simulink model "EmbeddedClosedLoop_Ard"  (Simulink 10.0)
settings: Solver=ode3  StartTime=0.0  StopTime=10.0  RelTol=1e-3
libraries: arduinolib x5, simulink x3
settings Model: Creator=deastman  LastModifiedBy=bhisma  ExtModeTrigDuration=2
settings DataIOCC: LimitDataPoints=on  SignalLoggingSaveFormat=ModelDataLogs
settings OptimizationCC: ExpressionDepthLimit=2147483647  LifeSpan=1  EfficientTunableParamExpr=on
settings DebuggingCC: FcnCallInpInsideContextMsg=warning  StateNameClashWarn=warning
settings HardwareCC: ProdBitPerInt=16  ProdBitPerPointer=16  ProdBitPerSizeT=16  ProdBitPerPtrDiffT=16  ProdIntDivRoundTo=Zero  ProdEndianess=LittleEndian  ProdWordSize=8  ProdHWDeviceType=Atmel->AVR
settings SFSimCC: MATLABDynamicMemAlloc=off
settings RTWCC: Description=Real-Time Toolbox  SystemTargetFile=realtime.tlc  GenerateMakefile=off  TemplateMakefile=realtime.tmf  RTWVerbose=off
settings CodeAppCC: CustomSymbolStrType=$N$R$M  InternalIdentifier=Classic
settings STFCustomTargetCC: TargetLibSuffix=.a  GenerateSampleERTMain=on  ERTCustomFileBanners=on  SupportNonInlinedSFcns=off  RemoveResetFunc=on  SupportVariableSizeSignals=on  MATLABClassNameForMDSCustomization=Simulink.SoftwareTarget.ERTCustomization  GRTInterface=off  SystemTargetFile=realtime.tlc
settings ERTTargetCC: MultiwordLength=2048  GenerateSampleERTMain=on  ParMdlRefBuildCompliant=off  CompOptLevelCompliant=off  ConcurrentExecutionCompliant=off  CombineOutputUpdateFcns=off  SupportContinuousTime=on  SupportVariableSizeSignals=on  ModelStepFunctionPrototypeControlCompliant=off  CPPClassGenCompliant=off  UseToolchainInfoCompliant=off  ERTSrcFileBannerTemplate=realtime_code_template.cgt  ERTHdrFileBannerTemplate=realtime_code_template.cgt  ERTDataSrcFileTemplate=realtime_code_template.cgt  ERTDataHdrFileTemplate=realtime_code_template.cgt  ERTCustomFileTemplate=realtime_file_process.tlc  ConvertIfToSwitch=off  SuppressUnreachableDefaultCases=off
settings ConfigComp: CovExternalEMLEnable=off
settings SimscapeCC: SimscapeNormalizeSystem=off
settings ConfigurationSet: Description=SimMechanics 2G
settings SettingsController: Description=Run on Hardware Dialog  TargetExtensionPlatform=Arduino Uno
settings MATStruct: Set_host_COM_port=[0.0]  COM_port_number=1  COM_port_baud_rate=115200  Enable_overrun_detection=[0.0]  Digital_output_to_set_on_overrun=13  Analog_input_reference_voltage=[0.0]  Serial0_baud_rate=9600

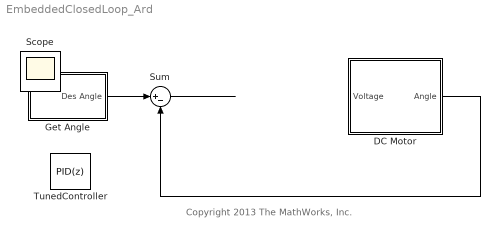
== system EmbeddedClosedLoop_Ard ==
  note: Copyright 2013 The MathWorks, Inc.
  DC Motor : Subsystem
  Get Angle : Subsystem
  Sum : Sum  Inputs=|+-
  TunedController : simulink/Continuous/PID Controller  Controller=PID  TimeDomain=Discrete-time  SampleTime=0.01  IntegratorMethod=Forward Euler  FilterMethod=Forward Euler  Form=Parallel  P=0.0932485816318116  I=0.0521328237727459  D=0.00709098323909587  N=12.2947610037998  InitialConditionSource=internal  InitialConditionForIntegrator=0  InitialConditionForFilter=0  ExternalReset=none  LimitOutput=on  UpperSaturationLimit=5  LowerSaturationLimit=-5  LinearizeAsGain=off  AntiWindupMode=clamping  Kb=1  TrackingMode=off  Kt=1  PParamMin=[]  PParamMax=[]  IParamMin=[]  IParamMax=[]  DParamMin=[]  DParamMax=[]  NParamMin=[]  NParamMax=[]  KbParamMin=[]  KbParamMax=[]  KtParamMin=[]  KtParamMax=[]  POutMin=[]  POutMax=[]  IOutMin=[]  IOutMax=[]  DOutMin=[]  DOutMax=[]  NOutMin=[]  NOutMax=[]  KbOutMin=[]  KbOutMax=[]  KtOutMin=[]  KtOutMax=[]  IntegratorOutMin=[]  IntegratorOutMax=[]  FilterOutMin=[]  FilterOutMax=[]  SumOutMin=[]  SumOutMax=[]  SumI1OutMin=[]  SumI1OutMax=[]  SumI2OutMin=[]  SumI2OutMax=[]  SumI3OutMin=[]  SumI3OutMax=[]  SumDOutMin=[]  SumDOutMax=[]  SaturationOutMin=[]  SaturationOutMax=[]  IntegratorContinuousStateAttributes=''  IntegratorStateMustResolveToSignalObject=off  IntegratorRTWStateStorageClass=Auto  FilterContinuousStateAttributes=''  FilterStateMustResolveToSignalObject=off  FilterRTWStateStorageClass=Auto
  Scope : Scope
  wires:
  DC Motor/1(Angle) -> Sum/2
  Get Angle/1(Des Angle) -> Sum/1
  Sum/1 -> ?
  ? -> DC Motor/1(Voltage)

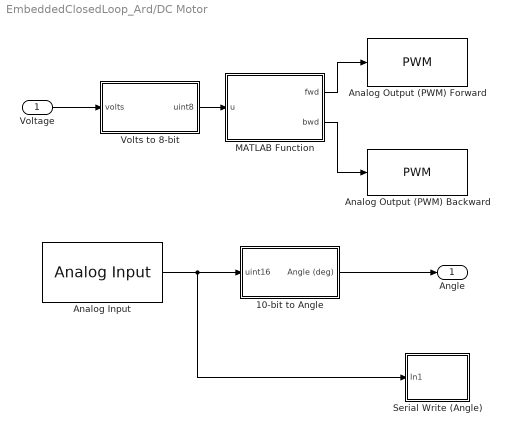
== system EmbeddedClosedLoop_Ard/DC Motor ==
  Voltage : Inport
  10-bit to Angle : Subsystem
  Analog Input : arduinolib/Analog Input  pinNumber=0  sampleTime=0.01
  Analog Output (PWM) Backward : arduinolib/PWM  pinNumber=11
  Analog Output (PWM) Forward : arduinolib/PWM  pinNumber=10
  MATLAB Function : MATLAB Function  TreatAsAtomicUnit=on
  Serial Write (Angle) : Subsystem
  Volts to 8-bit : Subsystem
  Angle : Outport
  wires:
  Volts to 8-bit/1(uint8) -> MATLAB Function/1(u)
  Voltage/1 -> Volts to 8-bit/1(volts)
  MATLAB Function/1(fwd) -> Analog Output (PWM) Forward/1
  MATLAB Function/2(bwd) -> Analog Output (PWM) Backward/1
  Analog Input/1 -> 10-bit to Angle/1(uint16), Serial Write (Angle)/1(In1)
  10-bit to Angle/1(Angle (deg)) -> Angle/1

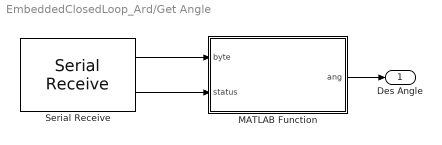
== system EmbeddedClosedLoop_Ard/Get Angle ==
  MATLAB Function : MATLAB Function  TreatAsAtomicUnit=on
  Serial Receive : arduinolib/Serial Receive  portNumber=0  showOutStatus=on  sampleTime=0.01
      settings: SourceProductName=Simulink Support Package for Arduino Hardware  SourceProductBaseCode=ARDUINO
  Des Angle : Outport
  wires:
  Serial Receive/1 -> MATLAB Function/1(byte)
  MATLAB Function/1(ang) -> Des Angle/1
  Serial Receive/2 -> MATLAB Function/2(status)

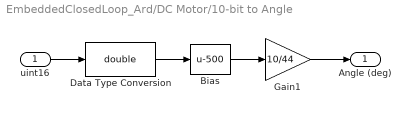
== system EmbeddedClosedLoop_Ard/DC Motor/10-bit to Angle ==
  uint16 : Inport
  Bias : Bias  Bias=-500
  Data Type Conversion : DataTypeConversion  OutDataTypeStr=double
  Gain1 : Gain  Gain=10/44
  Angle (deg) : Outport
  wires:
  Gain1/1 -> Angle (deg)/1
  uint16/1 -> Data Type Conversion/1
  Data Type Conversion/1 -> Bias/1
  Bias/1 -> Gain1/1

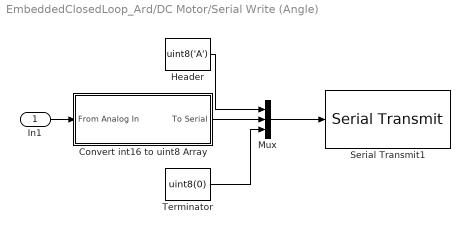
== system EmbeddedClosedLoop_Ard/DC Motor/Serial Write (Angle) ==
  In1 : Inport
  Convert int16 to uint8 Array : Subsystem
  Header : Constant  Value=uint8('A')
  Mux : Mux  Inputs=3
  Serial Transmit1 : arduinolib/Serial Transmit  portNumber=0
      settings: SourceProductName=Simulink Support Package for Arduino Hardware
  Terminator : Constant  Value=uint8(0)
  wires:
  Header/1 -> Mux/1
  Convert int16 to uint8 Array/1(To Serial) -> Mux/2
  Mux/1 -> Serial Transmit1/1
  Terminator/1 -> Mux/3
  In1/1 -> Convert int16 to uint8 Array/1(From Analog In)

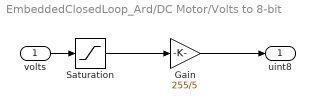
== system EmbeddedClosedLoop_Ard/DC Motor/Volts to 8-bit ==
  volts : Inport
  Gain : Gain  Gain=255/5  OutDataTypeStr=int16
  Saturation : Saturate  UpperLimit=5  LowerLimit=-5
  uint8 : Outport
  wires:
  Saturation/1 -> Gain/1
  Gain/1 -> uint8/1
  volts/1 -> Saturation/1

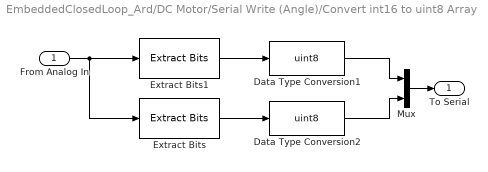
== system EmbeddedClosedLoop_Ard/DC Motor/Serial Write (Angle)/Convert int16 to uint8 Array ==
  From Analog In : Inport
  Data Type Conversion1 : DataTypeConversion  OutDataTypeStr=uint8  ConvertRealWorld=Stored Integer (SI)
  Data Type Conversion2 : DataTypeConversion  OutDataTypeStr=uint8  ConvertRealWorld=Stored Integer (SI)
  Extract Bits : simulink/Logic and Bit Operations/Extract Bits  bitsToExtract=Upper half  numBits=8  bitIdxRange=[0 7]  outScalingMode=Treat bit field as an integer
      settings: SourceProductName=Simulink
  Extract Bits1 : simulink/Logic and Bit Operations/Extract Bits  bitsToExtract=Lower half  numBits=8  bitIdxRange=[0 7]  outScalingMode=Treat bit field as an integer
      settings: SourceProductName=Simulink
  Mux : Mux  Inputs=2
  To Serial : Outport
  wires:
  From Analog In/1 -> Extract Bits/1, Extract Bits1/1
  Extract Bits1/1 -> Data Type Conversion1/1
  Extract Bits/1 -> Data Type Conversion2/1
  Data Type Conversion1/1 -> Mux/1
  Data Type Conversion2/1 -> Mux/2
  Mux/1 -> To Serial/1

== matlab function DC Motor/MATLAB Function ==
  data: u input double; fwd output double; bwd output double
function [fwd,bwd] = routeVoltage(u)
%#eml
if u>0
    fwd = uint8(u);
    bwd = uint8(0);
else
    fwd = uint8(0);
    bwd = uint8(-u);
end

== matlab function Get Angle/MATLAB Function ==
  data: byte input double; ang output double; status input double
function ang = passPosAngle(byte,status)
%#eml
persistent last

if isempty(last)
    last = 0;
end

if (byte >= 0 && status == 1)
    ang = double(byte)*(200/255)-100;
    last = ang;
else
    ang = last;
end
